simulink model "Table_airbus_v2"  (R2021b)
settings: Solver=VariableStepAuto  StartTime=0.0  StopTime=60*1.5  MaxStep=0.1  RelTol=0.01
undefined symbols (not defined in the file): X, Y, Z
libraries: sm_lib x907, fl_lib x68, nesl_utility x53, sdl_lib x10, simulink x7, ee_lib x7, slpidlib x6, simulink_extras x4
(part 18 of 18)

== system Table_airbus_v2/Modèle mécanique1/Table/table_1_RIGID/x15060_M_01002_Ens_cadre_Default_1_RIGID/x15060_NLM_Ens_guidage_Drylin_N_1_Default_1_RIGID/x15060_NLM_Palier_flottant_21230_2711_1_RIGID ==
  ReferenceFrame : sm_lib/Frames and Transforms/Reference Frame
  Solid : sm_lib/Body Elements/File Solid  ExtGeomFileName=15060-NLM-Palier flottant - 21230-2711_Défaut_sldprt.STL  UnitType=Custom  ExtGeomFileUnits=mm  StepReaderType=HEX  ExportConvexHullGeometry=off  InertiaType=Custom  Mass=0.0034336600000000003  MassUnits=kg  CenterOfMass=[20 6.8081300000000002 0.063214900000000004]  CenterOfMassUnits=mm  MomentsOfInertia=[0.14834700000000001 0.51841599999999999 0.39706900000000001]  MomentsOfInertiaUnits=kg*mm^2  ProductsOfInertia=[-0.00033843699999999997 0 0]  ProductsOfInertiaUnits=kg*mm^2  BasedOnType=Density  Density=1000  DensityUnits=kg/(m^3)  DoExposeReferenceFrame=on  SerializedFrames=<Frames/>  GraphicType=FromGeometry  MarkerShape=Sphere  MarkerSize=10  MarkerSizeUnits=m  GraphicVisPropType=SimpleVisualProperties  GraphicDiffuseColor=[0.792157 0.819608 0.933333]  GraphicSpecularColor=[0.5 0.5 0.5 1.0]  GraphicAmbientColor=[0.15 0.15 0.15 1.0]  GraphicEmissiveColor=[0.0 0.0 0.0 1.0]  GraphicShininess=75  GraphicOpacity=1
  F : PMIOPort  Side=Left
  connections:
  F/RConn1 -- ReferenceFrame/RConn1 -- Solid/RConn1

== system Table_airbus_v2/Modèle mécanique1/Table/table_1_RIGID/x15060_M_01002_Ens_cadre_Default_1_RIGID/x15060_NLM_Ens_guidage_Drylin_N_1_Default_1_RIGID/x15060_NLM_Palier_flottant_21230_2711_2_RIGID ==
  ReferenceFrame : sm_lib/Frames and Transforms/Reference Frame
  Solid : sm_lib/Body Elements/File Solid  ExtGeomFileName=15060-NLM-Palier flottant - 21230-2711_Défaut_sldprt.STL  UnitType=Custom  ExtGeomFileUnits=mm  StepReaderType=HEX  ExportConvexHullGeometry=off  InertiaType=Custom  Mass=0.0034336600000000003  MassUnits=kg  CenterOfMass=[20 6.8081300000000002 0.063214900000000004]  CenterOfMassUnits=mm  MomentsOfInertia=[0.14834700000000001 0.51841599999999999 0.39706900000000001]  MomentsOfInertiaUnits=kg*mm^2  ProductsOfInertia=[-0.00033843699999999997 0 0]  ProductsOfInertiaUnits=kg*mm^2  BasedOnType=Density  Density=1000  DensityUnits=kg/(m^3)  DoExposeReferenceFrame=on  SerializedFrames=<Frames/>  GraphicType=FromGeometry  MarkerShape=Sphere  MarkerSize=10  MarkerSizeUnits=m  GraphicVisPropType=SimpleVisualProperties  GraphicDiffuseColor=[0.792157 0.819608 0.933333]  GraphicSpecularColor=[0.5 0.5 0.5 1.0]  GraphicAmbientColor=[0.15 0.15 0.15 1.0]  GraphicEmissiveColor=[0.0 0.0 0.0 1.0]  GraphicShininess=75  GraphicOpacity=1
  F : PMIOPort  Side=Left
  connections:
  F/RConn1 -- ReferenceFrame/RConn1 -- Solid/RConn1

== system Table_airbus_v2/Modèle mécanique1/Table/table_1_RIGID/x15060_M_01002_Ens_cadre_Default_1_RIGID/x15060_NLM_Ens_guidage_Drylin_N_1_Default_1_RIGID/x15060_NLM_Palier_flottant_21230_2711_3_RIGID ==
  ReferenceFrame : sm_lib/Frames and Transforms/Reference Frame
  Solid : sm_lib/Body Elements/File Solid  ExtGeomFileName=15060-NLM-Palier flottant - 21230-2711_Défaut_sldprt.STL  UnitType=Custom  ExtGeomFileUnits=mm  StepReaderType=HEX  ExportConvexHullGeometry=off  InertiaType=Custom  Mass=0.0034336600000000003  MassUnits=kg  CenterOfMass=[20 6.8081300000000002 0.063214900000000004]  CenterOfMassUnits=mm  MomentsOfInertia=[0.14834700000000001 0.51841599999999999 0.39706900000000001]  MomentsOfInertiaUnits=kg*mm^2  ProductsOfInertia=[-0.00033843699999999997 0 0]  ProductsOfInertiaUnits=kg*mm^2  BasedOnType=Density  Density=1000  DensityUnits=kg/(m^3)  DoExposeReferenceFrame=on  SerializedFrames=<Frames/>  GraphicType=FromGeometry  MarkerShape=Sphere  MarkerSize=10  MarkerSizeUnits=m  GraphicVisPropType=SimpleVisualProperties  GraphicDiffuseColor=[0.792157 0.819608 0.933333]  GraphicSpecularColor=[0.5 0.5 0.5 1.0]  GraphicAmbientColor=[0.15 0.15 0.15 1.0]  GraphicEmissiveColor=[0.0 0.0 0.0 1.0]  GraphicShininess=75  GraphicOpacity=1
  F : PMIOPort  Side=Left
  connections:
  F/RConn1 -- ReferenceFrame/RConn1 -- Solid/RConn1

== system Table_airbus_v2/Modèle mécanique1/Table/table_1_RIGID/x15060_M_01002_Ens_cadre_Default_1_RIGID/x15060_NLM_Ens_guidage_Drylin_N_1_Default_1_RIGID/x15060_NLM_Palier_flottant_21230_2711_4_RIGID ==
  ReferenceFrame : sm_lib/Frames and Transforms/Reference Frame
  Solid : sm_lib/Body Elements/File Solid  ExtGeomFileName=15060-NLM-Palier flottant - 21230-2711_Défaut_sldprt.STL  UnitType=Custom  ExtGeomFileUnits=mm  StepReaderType=HEX  ExportConvexHullGeometry=off  InertiaType=Custom  Mass=0.0034336600000000003  MassUnits=kg  CenterOfMass=[20 6.8081300000000002 0.063214900000000004]  CenterOfMassUnits=mm  MomentsOfInertia=[0.14834700000000001 0.51841599999999999 0.39706900000000001]  MomentsOfInertiaUnits=kg*mm^2  ProductsOfInertia=[-0.00033843699999999997 0 0]  ProductsOfInertiaUnits=kg*mm^2  BasedOnType=Density  Density=1000  DensityUnits=kg/(m^3)  DoExposeReferenceFrame=on  SerializedFrames=<Frames/>  GraphicType=FromGeometry  MarkerShape=Sphere  MarkerSize=10  MarkerSizeUnits=m  GraphicVisPropType=SimpleVisualProperties  GraphicDiffuseColor=[0.792157 0.819608 0.933333]  GraphicSpecularColor=[0.5 0.5 0.5 1.0]  GraphicAmbientColor=[0.15 0.15 0.15 1.0]  GraphicEmissiveColor=[0.0 0.0 0.0 1.0]  GraphicShininess=75  GraphicOpacity=1
  F : PMIOPort  Side=Left
  connections:
  F/RConn1 -- ReferenceFrame/RConn1 -- Solid/RConn1

== system Table_airbus_v2/Modèle mécanique1/Table/table_1_RIGID/x15060_M_01002_Ens_cadre_Default_1_RIGID/x15060_NLM_Ens_guidage_Drylin_N_1_Default_1_RIGID/x15060_NLM_Rail_21230_2730_X_Lgr_1_RIGID ==
  ReferenceFrame : sm_lib/Frames and Transforms/Reference Frame
  Solid : sm_lib/Body Elements/File Solid  ExtGeomFileName=15060-NLM-Rail - 21230-2730 X Lgr._Défaut_sldprt.STL  UnitType=Custom  ExtGeomFileUnits=mm  StepReaderType=HEX  ExportConvexHullGeometry=off  InertiaType=Custom  Mass=0.068416199999999996  MassUnits=kg  CenterOfMass=[390 3.0880299999999998 0]  CenterOfMassUnits=mm  MomentsOfInertia=[4.6660399999999997 2573.8499999999999 2569.9400000000001]  MomentsOfInertiaUnits=kg*mm^2  ProductsOfInertia=[0 0 0]  ProductsOfInertiaUnits=kg*mm^2  BasedOnType=Density  Density=1000  DensityUnits=kg/(m^3)  DoExposeReferenceFrame=on  SerializedFrames=<Frames/>  GraphicType=FromGeometry  MarkerShape=Sphere  MarkerSize=10  MarkerSizeUnits=m  GraphicVisPropType=SimpleVisualProperties  GraphicDiffuseColor=[0.792157 0.819608 0.933333]  GraphicSpecularColor=[0.5 0.5 0.5 1.0]  GraphicAmbientColor=[0.15 0.15 0.15 1.0]  GraphicEmissiveColor=[0.0 0.0 0.0 1.0]  GraphicShininess=75  GraphicOpacity=1
  F : PMIOPort  Side=Left
  connections:
  F/RConn1 -- ReferenceFrame/RConn1 -- Solid/RConn1

== system Table_airbus_v2/Modèle mécanique1/Table/table_1_RIGID/x15060_M_01002_Ens_cadre_Default_1_RIGID/x15060_NLM_Ens_guidage_Drylin_N_1_Default_2_RIGID/x15060_NLM_Palier_flottant_21230_2711_1_RIGID ==
  ReferenceFrame : sm_lib/Frames and Transforms/Reference Frame
  Solid : sm_lib/Body Elements/File Solid  ExtGeomFileName=15060-NLM-Palier flottant - 21230-2711_Défaut_sldprt.STL  UnitType=Custom  ExtGeomFileUnits=mm  StepReaderType=HEX  ExportConvexHullGeometry=off  InertiaType=Custom  Mass=0.0034336600000000003  MassUnits=kg  CenterOfMass=[20 6.8081300000000002 0.063214900000000004]  CenterOfMassUnits=mm  MomentsOfInertia=[0.14834700000000001 0.51841599999999999 0.39706900000000001]  MomentsOfInertiaUnits=kg*mm^2  ProductsOfInertia=[-0.00033843699999999997 0 0]  ProductsOfInertiaUnits=kg*mm^2  BasedOnType=Density  Density=1000  DensityUnits=kg/(m^3)  DoExposeReferenceFrame=on  SerializedFrames=<Frames/>  GraphicType=FromGeometry  MarkerShape=Sphere  MarkerSize=10  MarkerSizeUnits=m  GraphicVisPropType=SimpleVisualProperties  GraphicDiffuseColor=[0.792157 0.819608 0.933333]  GraphicSpecularColor=[0.5 0.5 0.5 1.0]  GraphicAmbientColor=[0.15 0.15 0.15 1.0]  GraphicEmissiveColor=[0.0 0.0 0.0 1.0]  GraphicShininess=75  GraphicOpacity=1
  F : PMIOPort  Side=Left
  connections:
  F/RConn1 -- ReferenceFrame/RConn1 -- Solid/RConn1

== system Table_airbus_v2/Modèle mécanique1/Table/table_1_RIGID/x15060_M_01002_Ens_cadre_Default_1_RIGID/x15060_NLM_Ens_guidage_Drylin_N_1_Default_2_RIGID/x15060_NLM_Palier_flottant_21230_2711_2_RIGID ==
  ReferenceFrame : sm_lib/Frames and Transforms/Reference Frame
  Solid : sm_lib/Body Elements/File Solid  ExtGeomFileName=15060-NLM-Palier flottant - 21230-2711_Défaut_sldprt.STL  UnitType=Custom  ExtGeomFileUnits=mm  StepReaderType=HEX  ExportConvexHullGeometry=off  InertiaType=Custom  Mass=0.0034336600000000003  MassUnits=kg  CenterOfMass=[20 6.8081300000000002 0.063214900000000004]  CenterOfMassUnits=mm  MomentsOfInertia=[0.14834700000000001 0.51841599999999999 0.39706900000000001]  MomentsOfInertiaUnits=kg*mm^2  ProductsOfInertia=[-0.00033843699999999997 0 0]  ProductsOfInertiaUnits=kg*mm^2  BasedOnType=Density  Density=1000  DensityUnits=kg/(m^3)  DoExposeReferenceFrame=on  SerializedFrames=<Frames/>  GraphicType=FromGeometry  MarkerShape=Sphere  MarkerSize=10  MarkerSizeUnits=m  GraphicVisPropType=SimpleVisualProperties  GraphicDiffuseColor=[0.792157 0.819608 0.933333]  GraphicSpecularColor=[0.5 0.5 0.5 1.0]  GraphicAmbientColor=[0.15 0.15 0.15 1.0]  GraphicEmissiveColor=[0.0 0.0 0.0 1.0]  GraphicShininess=75  GraphicOpacity=1
  F : PMIOPort  Side=Left
  connections:
  F/RConn1 -- ReferenceFrame/RConn1 -- Solid/RConn1

== system Table_airbus_v2/Modèle mécanique1/Table/table_1_RIGID/x15060_M_01002_Ens_cadre_Default_1_RIGID/x15060_NLM_Ens_guidage_Drylin_N_1_Default_2_RIGID/x15060_NLM_Palier_flottant_21230_2711_3_RIGID ==
  ReferenceFrame : sm_lib/Frames and Transforms/Reference Frame
  Solid : sm_lib/Body Elements/File Solid  ExtGeomFileName=15060-NLM-Palier flottant - 21230-2711_Défaut_sldprt.STL  UnitType=Custom  ExtGeomFileUnits=mm  StepReaderType=HEX  ExportConvexHullGeometry=off  InertiaType=Custom  Mass=0.0034336600000000003  MassUnits=kg  CenterOfMass=[20 6.8081300000000002 0.063214900000000004]  CenterOfMassUnits=mm  MomentsOfInertia=[0.14834700000000001 0.51841599999999999 0.39706900000000001]  MomentsOfInertiaUnits=kg*mm^2  ProductsOfInertia=[-0.00033843699999999997 0 0]  ProductsOfInertiaUnits=kg*mm^2  BasedOnType=Density  Density=1000  DensityUnits=kg/(m^3)  DoExposeReferenceFrame=on  SerializedFrames=<Frames/>  GraphicType=FromGeometry  MarkerShape=Sphere  MarkerSize=10  MarkerSizeUnits=m  GraphicVisPropType=SimpleVisualProperties  GraphicDiffuseColor=[0.792157 0.819608 0.933333]  GraphicSpecularColor=[0.5 0.5 0.5 1.0]  GraphicAmbientColor=[0.15 0.15 0.15 1.0]  GraphicEmissiveColor=[0.0 0.0 0.0 1.0]  GraphicShininess=75  GraphicOpacity=1
  F : PMIOPort  Side=Left
  connections:
  F/RConn1 -- ReferenceFrame/RConn1 -- Solid/RConn1

== system Table_airbus_v2/Modèle mécanique1/Table/table_1_RIGID/x15060_M_01002_Ens_cadre_Default_1_RIGID/x15060_NLM_Ens_guidage_Drylin_N_1_Default_2_RIGID/x15060_NLM_Palier_flottant_21230_2711_4_RIGID ==
  ReferenceFrame : sm_lib/Frames and Transforms/Reference Frame
  Solid : sm_lib/Body Elements/File Solid  ExtGeomFileName=15060-NLM-Palier flottant - 21230-2711_Défaut_sldprt.STL  UnitType=Custom  ExtGeomFileUnits=mm  StepReaderType=HEX  ExportConvexHullGeometry=off  InertiaType=Custom  Mass=0.0034336600000000003  MassUnits=kg  CenterOfMass=[20 6.8081300000000002 0.063214900000000004]  CenterOfMassUnits=mm  MomentsOfInertia=[0.14834700000000001 0.51841599999999999 0.39706900000000001]  MomentsOfInertiaUnits=kg*mm^2  ProductsOfInertia=[-0.00033843699999999997 0 0]  ProductsOfInertiaUnits=kg*mm^2  BasedOnType=Density  Density=1000  DensityUnits=kg/(m^3)  DoExposeReferenceFrame=on  SerializedFrames=<Frames/>  GraphicType=FromGeometry  MarkerShape=Sphere  MarkerSize=10  MarkerSizeUnits=m  GraphicVisPropType=SimpleVisualProperties  GraphicDiffuseColor=[0.792157 0.819608 0.933333]  GraphicSpecularColor=[0.5 0.5 0.5 1.0]  GraphicAmbientColor=[0.15 0.15 0.15 1.0]  GraphicEmissiveColor=[0.0 0.0 0.0 1.0]  GraphicShininess=75  GraphicOpacity=1
  F : PMIOPort  Side=Left
  connections:
  F/RConn1 -- ReferenceFrame/RConn1 -- Solid/RConn1

== system Table_airbus_v2/Modèle mécanique1/Table/table_1_RIGID/x15060_M_01002_Ens_cadre_Default_1_RIGID/x15060_NLM_Ens_guidage_Drylin_N_1_Default_2_RIGID/x15060_NLM_Rail_21230_2730_X_Lgr_1_RIGID ==
  ReferenceFrame : sm_lib/Frames and Transforms/Reference Frame
  Solid : sm_lib/Body Elements/File Solid  ExtGeomFileName=15060-NLM-Rail - 21230-2730 X Lgr._Défaut_sldprt.STL  UnitType=Custom  ExtGeomFileUnits=mm  StepReaderType=HEX  ExportConvexHullGeometry=off  InertiaType=Custom  Mass=0.068416199999999996  MassUnits=kg  CenterOfMass=[390 3.0880299999999998 0]  CenterOfMassUnits=mm  MomentsOfInertia=[4.6660399999999997 2573.8499999999999 2569.9400000000001]  MomentsOfInertiaUnits=kg*mm^2  ProductsOfInertia=[0 0 0]  ProductsOfInertiaUnits=kg*mm^2  BasedOnType=Density  Density=1000  DensityUnits=kg/(m^3)  DoExposeReferenceFrame=on  SerializedFrames=<Frames/>  GraphicType=FromGeometry  MarkerShape=Sphere  MarkerSize=10  MarkerSizeUnits=m  GraphicVisPropType=SimpleVisualProperties  GraphicDiffuseColor=[0.792157 0.819608 0.933333]  GraphicSpecularColor=[0.5 0.5 0.5 1.0]  GraphicAmbientColor=[0.15 0.15 0.15 1.0]  GraphicEmissiveColor=[0.0 0.0 0.0 1.0]  GraphicShininess=75  GraphicOpacity=1
  F : PMIOPort  Side=Left
  connections:
  F/RConn1 -- ReferenceFrame/RConn1 -- Solid/RConn1

== system Table_airbus_v2/Modèle mécanique1/Table/table_1_RIGID/x15060_M_01002_Ens_cadre_Default_1_RIGID/x15060_NLM_Ens_guidage_Drylin_N_1_Default_3_RIGID/x15060_NLM_Palier_flottant_21230_2711_1_RIGID ==
  ReferenceFrame : sm_lib/Frames and Transforms/Reference Frame
  Solid : sm_lib/Body Elements/File Solid  ExtGeomFileName=15060-NLM-Palier flottant - 21230-2711_Défaut_sldprt.STL  UnitType=Custom  ExtGeomFileUnits=mm  StepReaderType=HEX  ExportConvexHullGeometry=off  InertiaType=Custom  Mass=0.0034336600000000003  MassUnits=kg  CenterOfMass=[20 6.8081300000000002 0.063214900000000004]  CenterOfMassUnits=mm  MomentsOfInertia=[0.14834700000000001 0.51841599999999999 0.39706900000000001]  MomentsOfInertiaUnits=kg*mm^2  ProductsOfInertia=[-0.00033843699999999997 0 0]  ProductsOfInertiaUnits=kg*mm^2  BasedOnType=Density  Density=1000  DensityUnits=kg/(m^3)  DoExposeReferenceFrame=on  SerializedFrames=<Frames/>  GraphicType=FromGeometry  MarkerShape=Sphere  MarkerSize=10  MarkerSizeUnits=m  GraphicVisPropType=SimpleVisualProperties  GraphicDiffuseColor=[0.792157 0.819608 0.933333]  GraphicSpecularColor=[0.5 0.5 0.5 1.0]  GraphicAmbientColor=[0.15 0.15 0.15 1.0]  GraphicEmissiveColor=[0.0 0.0 0.0 1.0]  GraphicShininess=75  GraphicOpacity=1
  F : PMIOPort  Side=Left
  connections:
  F/RConn1 -- ReferenceFrame/RConn1 -- Solid/RConn1

== system Table_airbus_v2/Modèle mécanique1/Table/table_1_RIGID/x15060_M_01002_Ens_cadre_Default_1_RIGID/x15060_NLM_Ens_guidage_Drylin_N_1_Default_3_RIGID/x15060_NLM_Palier_flottant_21230_2711_2_RIGID ==
  ReferenceFrame : sm_lib/Frames and Transforms/Reference Frame
  Solid : sm_lib/Body Elements/File Solid  ExtGeomFileName=15060-NLM-Palier flottant - 21230-2711_Défaut_sldprt.STL  UnitType=Custom  ExtGeomFileUnits=mm  StepReaderType=HEX  ExportConvexHullGeometry=off  InertiaType=Custom  Mass=0.0034336600000000003  MassUnits=kg  CenterOfMass=[20 6.8081300000000002 0.063214900000000004]  CenterOfMassUnits=mm  MomentsOfInertia=[0.14834700000000001 0.51841599999999999 0.39706900000000001]  MomentsOfInertiaUnits=kg*mm^2  ProductsOfInertia=[-0.00033843699999999997 0 0]  ProductsOfInertiaUnits=kg*mm^2  BasedOnType=Density  Density=1000  DensityUnits=kg/(m^3)  DoExposeReferenceFrame=on  SerializedFrames=<Frames/>  GraphicType=FromGeometry  MarkerShape=Sphere  MarkerSize=10  MarkerSizeUnits=m  GraphicVisPropType=SimpleVisualProperties  GraphicDiffuseColor=[0.792157 0.819608 0.933333]  GraphicSpecularColor=[0.5 0.5 0.5 1.0]  GraphicAmbientColor=[0.15 0.15 0.15 1.0]  GraphicEmissiveColor=[0.0 0.0 0.0 1.0]  GraphicShininess=75  GraphicOpacity=1
  F : PMIOPort  Side=Left
  connections:
  F/RConn1 -- ReferenceFrame/RConn1 -- Solid/RConn1

== system Table_airbus_v2/Modèle mécanique1/Table/table_1_RIGID/x15060_M_01002_Ens_cadre_Default_1_RIGID/x15060_NLM_Ens_guidage_Drylin_N_1_Default_3_RIGID/x15060_NLM_Palier_flottant_21230_2711_3_RIGID ==
  ReferenceFrame : sm_lib/Frames and Transforms/Reference Frame
  Solid : sm_lib/Body Elements/File Solid  ExtGeomFileName=15060-NLM-Palier flottant - 21230-2711_Défaut_sldprt.STL  UnitType=Custom  ExtGeomFileUnits=mm  StepReaderType=HEX  ExportConvexHullGeometry=off  InertiaType=Custom  Mass=0.0034336600000000003  MassUnits=kg  CenterOfMass=[20 6.8081300000000002 0.063214900000000004]  CenterOfMassUnits=mm  MomentsOfInertia=[0.14834700000000001 0.51841599999999999 0.39706900000000001]  MomentsOfInertiaUnits=kg*mm^2  ProductsOfInertia=[-0.00033843699999999997 0 0]  ProductsOfInertiaUnits=kg*mm^2  BasedOnType=Density  Density=1000  DensityUnits=kg/(m^3)  DoExposeReferenceFrame=on  SerializedFrames=<Frames/>  GraphicType=FromGeometry  MarkerShape=Sphere  MarkerSize=10  MarkerSizeUnits=m  GraphicVisPropType=SimpleVisualProperties  GraphicDiffuseColor=[0.792157 0.819608 0.933333]  GraphicSpecularColor=[0.5 0.5 0.5 1.0]  GraphicAmbientColor=[0.15 0.15 0.15 1.0]  GraphicEmissiveColor=[0.0 0.0 0.0 1.0]  GraphicShininess=75  GraphicOpacity=1
  F : PMIOPort  Side=Left
  connections:
  F/RConn1 -- ReferenceFrame/RConn1 -- Solid/RConn1

== system Table_airbus_v2/Modèle mécanique1/Table/table_1_RIGID/x15060_M_01002_Ens_cadre_Default_1_RIGID/x15060_NLM_Ens_guidage_Drylin_N_1_Default_3_RIGID/x15060_NLM_Palier_flottant_21230_2711_4_RIGID ==
  ReferenceFrame : sm_lib/Frames and Transforms/Reference Frame
  Solid : sm_lib/Body Elements/File Solid  ExtGeomFileName=15060-NLM-Palier flottant - 21230-2711_Défaut_sldprt.STL  UnitType=Custom  ExtGeomFileUnits=mm  StepReaderType=HEX  ExportConvexHullGeometry=off  InertiaType=Custom  Mass=0.0034336600000000003  MassUnits=kg  CenterOfMass=[20 6.8081300000000002 0.063214900000000004]  CenterOfMassUnits=mm  MomentsOfInertia=[0.14834700000000001 0.51841599999999999 0.39706900000000001]  MomentsOfInertiaUnits=kg*mm^2  ProductsOfInertia=[-0.00033843699999999997 0 0]  ProductsOfInertiaUnits=kg*mm^2  BasedOnType=Density  Density=1000  DensityUnits=kg/(m^3)  DoExposeReferenceFrame=on  SerializedFrames=<Frames/>  GraphicType=FromGeometry  MarkerShape=Sphere  MarkerSize=10  MarkerSizeUnits=m  GraphicVisPropType=SimpleVisualProperties  GraphicDiffuseColor=[0.792157 0.819608 0.933333]  GraphicSpecularColor=[0.5 0.5 0.5 1.0]  GraphicAmbientColor=[0.15 0.15 0.15 1.0]  GraphicEmissiveColor=[0.0 0.0 0.0 1.0]  GraphicShininess=75  GraphicOpacity=1
  F : PMIOPort  Side=Left
  connections:
  F/RConn1 -- ReferenceFrame/RConn1 -- Solid/RConn1

== system Table_airbus_v2/Modèle mécanique1/Table/table_1_RIGID/x15060_M_01002_Ens_cadre_Default_1_RIGID/x15060_NLM_Ens_guidage_Drylin_N_1_Default_3_RIGID/x15060_NLM_Rail_21230_2730_X_Lgr_1_RIGID ==
  ReferenceFrame : sm_lib/Frames and Transforms/Reference Frame
  Solid : sm_lib/Body Elements/File Solid  ExtGeomFileName=15060-NLM-Rail - 21230-2730 X Lgr._Défaut_sldprt.STL  UnitType=Custom  ExtGeomFileUnits=mm  StepReaderType=HEX  ExportConvexHullGeometry=off  InertiaType=Custom  Mass=0.068416199999999996  MassUnits=kg  CenterOfMass=[390 3.0880299999999998 0]  CenterOfMassUnits=mm  MomentsOfInertia=[4.6660399999999997 2573.8499999999999 2569.9400000000001]  MomentsOfInertiaUnits=kg*mm^2  ProductsOfInertia=[0 0 0]  ProductsOfInertiaUnits=kg*mm^2  BasedOnType=Density  Density=1000  DensityUnits=kg/(m^3)  DoExposeReferenceFrame=on  SerializedFrames=<Frames/>  GraphicType=FromGeometry  MarkerShape=Sphere  MarkerSize=10  MarkerSizeUnits=m  GraphicVisPropType=SimpleVisualProperties  GraphicDiffuseColor=[0.792157 0.819608 0.933333]  GraphicSpecularColor=[0.5 0.5 0.5 1.0]  GraphicAmbientColor=[0.15 0.15 0.15 1.0]  GraphicEmissiveColor=[0.0 0.0 0.0 1.0]  GraphicShininess=75  GraphicOpacity=1
  F : PMIOPort  Side=Left
  connections:
  F/RConn1 -- ReferenceFrame/RConn1 -- Solid/RConn1

== system Table_airbus_v2/Modèle mécanique1/Table/table_1_RIGID/x15060_M_01002_Ens_cadre_Default_1_RIGID/x15060_NLM_Ens_guidage_Drylin_N_1_Default_4_RIGID/x15060_NLM_Palier_flottant_21230_2711_1_RIGID ==
  ReferenceFrame : sm_lib/Frames and Transforms/Reference Frame
  Solid : sm_lib/Body Elements/File Solid  ExtGeomFileName=15060-NLM-Palier flottant - 21230-2711_Défaut_sldprt.STL  UnitType=Custom  ExtGeomFileUnits=mm  StepReaderType=HEX  ExportConvexHullGeometry=off  InertiaType=Custom  Mass=0.0034336600000000003  MassUnits=kg  CenterOfMass=[20 6.8081300000000002 0.063214900000000004]  CenterOfMassUnits=mm  MomentsOfInertia=[0.14834700000000001 0.51841599999999999 0.39706900000000001]  MomentsOfInertiaUnits=kg*mm^2  ProductsOfInertia=[-0.00033843699999999997 0 0]  ProductsOfInertiaUnits=kg*mm^2  BasedOnType=Density  Density=1000  DensityUnits=kg/(m^3)  DoExposeReferenceFrame=on  SerializedFrames=<Frames/>  GraphicType=FromGeometry  MarkerShape=Sphere  MarkerSize=10  MarkerSizeUnits=m  GraphicVisPropType=SimpleVisualProperties  GraphicDiffuseColor=[0.792157 0.819608 0.933333]  GraphicSpecularColor=[0.5 0.5 0.5 1.0]  GraphicAmbientColor=[0.15 0.15 0.15 1.0]  GraphicEmissiveColor=[0.0 0.0 0.0 1.0]  GraphicShininess=75  GraphicOpacity=1
  F : PMIOPort  Side=Left
  connections:
  F/RConn1 -- ReferenceFrame/RConn1 -- Solid/RConn1

== system Table_airbus_v2/Modèle mécanique1/Table/table_1_RIGID/x15060_M_01002_Ens_cadre_Default_1_RIGID/x15060_NLM_Ens_guidage_Drylin_N_1_Default_4_RIGID/x15060_NLM_Palier_flottant_21230_2711_2_RIGID ==
  ReferenceFrame : sm_lib/Frames and Transforms/Reference Frame
  Solid : sm_lib/Body Elements/File Solid  ExtGeomFileName=15060-NLM-Palier flottant - 21230-2711_Défaut_sldprt.STL  UnitType=Custom  ExtGeomFileUnits=mm  StepReaderType=HEX  ExportConvexHullGeometry=off  InertiaType=Custom  Mass=0.0034336600000000003  MassUnits=kg  CenterOfMass=[20 6.8081300000000002 0.063214900000000004]  CenterOfMassUnits=mm  MomentsOfInertia=[0.14834700000000001 0.51841599999999999 0.39706900000000001]  MomentsOfInertiaUnits=kg*mm^2  ProductsOfInertia=[-0.00033843699999999997 0 0]  ProductsOfInertiaUnits=kg*mm^2  BasedOnType=Density  Density=1000  DensityUnits=kg/(m^3)  DoExposeReferenceFrame=on  SerializedFrames=<Frames/>  GraphicType=FromGeometry  MarkerShape=Sphere  MarkerSize=10  MarkerSizeUnits=m  GraphicVisPropType=SimpleVisualProperties  GraphicDiffuseColor=[0.792157 0.819608 0.933333]  GraphicSpecularColor=[0.5 0.5 0.5 1.0]  GraphicAmbientColor=[0.15 0.15 0.15 1.0]  GraphicEmissiveColor=[0.0 0.0 0.0 1.0]  GraphicShininess=75  GraphicOpacity=1
  F : PMIOPort  Side=Left
  connections:
  F/RConn1 -- ReferenceFrame/RConn1 -- Solid/RConn1

== system Table_airbus_v2/Modèle mécanique1/Table/table_1_RIGID/x15060_M_01002_Ens_cadre_Default_1_RIGID/x15060_NLM_Ens_guidage_Drylin_N_1_Default_4_RIGID/x15060_NLM_Palier_flottant_21230_2711_3_RIGID ==
  ReferenceFrame : sm_lib/Frames and Transforms/Reference Frame
  Solid : sm_lib/Body Elements/File Solid  ExtGeomFileName=15060-NLM-Palier flottant - 21230-2711_Défaut_sldprt.STL  UnitType=Custom  ExtGeomFileUnits=mm  StepReaderType=HEX  ExportConvexHullGeometry=off  InertiaType=Custom  Mass=0.0034336600000000003  MassUnits=kg  CenterOfMass=[20 6.8081300000000002 0.063214900000000004]  CenterOfMassUnits=mm  MomentsOfInertia=[0.14834700000000001 0.51841599999999999 0.39706900000000001]  MomentsOfInertiaUnits=kg*mm^2  ProductsOfInertia=[-0.00033843699999999997 0 0]  ProductsOfInertiaUnits=kg*mm^2  BasedOnType=Density  Density=1000  DensityUnits=kg/(m^3)  DoExposeReferenceFrame=on  SerializedFrames=<Frames/>  GraphicType=FromGeometry  MarkerShape=Sphere  MarkerSize=10  MarkerSizeUnits=m  GraphicVisPropType=SimpleVisualProperties  GraphicDiffuseColor=[0.792157 0.819608 0.933333]  GraphicSpecularColor=[0.5 0.5 0.5 1.0]  GraphicAmbientColor=[0.15 0.15 0.15 1.0]  GraphicEmissiveColor=[0.0 0.0 0.0 1.0]  GraphicShininess=75  GraphicOpacity=1
  F : PMIOPort  Side=Left
  connections:
  F/RConn1 -- ReferenceFrame/RConn1 -- Solid/RConn1

== system Table_airbus_v2/Modèle mécanique1/Table/table_1_RIGID/x15060_M_01002_Ens_cadre_Default_1_RIGID/x15060_NLM_Ens_guidage_Drylin_N_1_Default_4_RIGID/x15060_NLM_Palier_flottant_21230_2711_4_RIGID ==
  ReferenceFrame : sm_lib/Frames and Transforms/Reference Frame
  Solid : sm_lib/Body Elements/File Solid  ExtGeomFileName=15060-NLM-Palier flottant - 21230-2711_Défaut_sldprt.STL  UnitType=Custom  ExtGeomFileUnits=mm  StepReaderType=HEX  ExportConvexHullGeometry=off  InertiaType=Custom  Mass=0.0034336600000000003  MassUnits=kg  CenterOfMass=[20 6.8081300000000002 0.063214900000000004]  CenterOfMassUnits=mm  MomentsOfInertia=[0.14834700000000001 0.51841599999999999 0.39706900000000001]  MomentsOfInertiaUnits=kg*mm^2  ProductsOfInertia=[-0.00033843699999999997 0 0]  ProductsOfInertiaUnits=kg*mm^2  BasedOnType=Density  Density=1000  DensityUnits=kg/(m^3)  DoExposeReferenceFrame=on  SerializedFrames=<Frames/>  GraphicType=FromGeometry  MarkerShape=Sphere  MarkerSize=10  MarkerSizeUnits=m  GraphicVisPropType=SimpleVisualProperties  GraphicDiffuseColor=[0.792157 0.819608 0.933333]  GraphicSpecularColor=[0.5 0.5 0.5 1.0]  GraphicAmbientColor=[0.15 0.15 0.15 1.0]  GraphicEmissiveColor=[0.0 0.0 0.0 1.0]  GraphicShininess=75  GraphicOpacity=1
  F : PMIOPort  Side=Left
  connections:
  F/RConn1 -- ReferenceFrame/RConn1 -- Solid/RConn1

== system Table_airbus_v2/Modèle mécanique1/Table/table_1_RIGID/x15060_M_01002_Ens_cadre_Default_1_RIGID/x15060_NLM_Ens_guidage_Drylin_N_1_Default_4_RIGID/x15060_NLM_Rail_21230_2730_X_Lgr_1_RIGID ==
  ReferenceFrame : sm_lib/Frames and Transforms/Reference Frame
  Solid : sm_lib/Body Elements/File Solid  ExtGeomFileName=15060-NLM-Rail - 21230-2730 X Lgr._Défaut_sldprt.STL  UnitType=Custom  ExtGeomFileUnits=mm  StepReaderType=HEX  ExportConvexHullGeometry=off  InertiaType=Custom  Mass=0.068416199999999996  MassUnits=kg  CenterOfMass=[390 3.0880299999999998 0]  CenterOfMassUnits=mm  MomentsOfInertia=[4.6660399999999997 2573.8499999999999 2569.9400000000001]  MomentsOfInertiaUnits=kg*mm^2  ProductsOfInertia=[0 0 0]  ProductsOfInertiaUnits=kg*mm^2  BasedOnType=Density  Density=1000  DensityUnits=kg/(m^3)  DoExposeReferenceFrame=on  SerializedFrames=<Frames/>  GraphicType=FromGeometry  MarkerShape=Sphere  MarkerSize=10  MarkerSizeUnits=m  GraphicVisPropType=SimpleVisualProperties  GraphicDiffuseColor=[0.792157 0.819608 0.933333]  GraphicSpecularColor=[0.5 0.5 0.5 1.0]  GraphicAmbientColor=[0.15 0.15 0.15 1.0]  GraphicEmissiveColor=[0.0 0.0 0.0 1.0]  GraphicShininess=75  GraphicOpacity=1
  F : PMIOPort  Side=Left
  connections:
  F/RConn1 -- ReferenceFrame/RConn1 -- Solid/RConn1

== system Table_airbus_v2/Modèle mécanique1/Table/table_1_RIGID/x15060_M_01014_Ens_plateau_Default_1_RIGID/x15060_M_01003_Ens_structure_plateau_Default_1_RIGID/x15060_ITEM_Kit_Equerre_8_40x40_Zn_0_0_411_15_AA_DEFAULT_1_RIGI ==
  ReferenceFrame : sm_lib/Frames and Transforms/Reference Frame
  Solid : sm_lib/Body Elements/File Solid  ExtGeomFileName=15060-ITEM-Kit Equerre 8 40x40 Zn - 0.0.411.15_AA - DEFAULT_Défaut_sldprt.STL  UnitType=Custom  ExtGeomFileUnits=mm  StepReaderType=HEX  ExportConvexHullGeometry=off  InertiaType=Custom  Mass=0.010278799999999999  MassUnits=kg  CenterOfMass=[11.6701 11.6701 0]  CenterOfMassUnits=mm  MomentsOfInertia=[3.3914200000000001 3.3914200000000001 2.6288999999999998]  MomentsOfInertiaUnits=kg*mm^2  ProductsOfInertia=[0 0 -0.71321800000000002]  ProductsOfInertiaUnits=kg*mm^2  BasedOnType=Density  Density=1000  DensityUnits=kg/(m^3)  DoExposeReferenceFrame=on  SerializedFrames=<Frames/>  GraphicType=FromGeometry  MarkerShape=Sphere  MarkerSize=10  MarkerSizeUnits=m  GraphicVisPropType=SimpleVisualProperties  GraphicDiffuseColor=[0.792157 0.819608 0.933333]  GraphicSpecularColor=[0.5 0.5 0.5 1.0]  GraphicAmbientColor=[0.15 0.15 0.15 1.0]  GraphicEmissiveColor=[0.0 0.0 0.0 1.0]  GraphicShininess=75  GraphicOpacity=1
  F : PMIOPort  Side=Left
  connections:
  F/RConn1 -- ReferenceFrame/RConn1 -- Solid/RConn1

== system Table_airbus_v2/Modèle mécanique1/Table/table_1_RIGID/x15060_M_01014_Ens_plateau_Default_1_RIGID/x15060_M_01003_Ens_structure_plateau_Default_1_RIGID/x15060_ITEM_Kit_Equerre_8_80x80_Zn_0_0_411_32_AA_DEFAULT_1_RIGI ==
  ReferenceFrame : sm_lib/Frames and Transforms/Reference Frame
  Solid : sm_lib/Body Elements/File Solid  ExtGeomFileName=15060-ITEM-Kit Equerre 8 80x80 Zn - 0.0.411.32_AA - DEFAULT_Défaut_sldprt.STL  UnitType=Custom  ExtGeomFileUnits=mm  StepReaderType=HEX  ExportConvexHullGeometry=off  InertiaType=Custom  Mass=0.078431600000000004  MassUnits=kg  CenterOfMass=[23.9558 23.9558 0]  CenterOfMassUnits=mm  MomentsOfInertia=[57.169000000000004 57.169000000000004 76.38539999999999]  MomentsOfInertiaUnits=kg*mm^2  ProductsOfInertia=[0 0 -20.189700000000002]  ProductsOfInertiaUnits=kg*mm^2  BasedOnType=Density  Density=1000  DensityUnits=kg/(m^3)  DoExposeReferenceFrame=on  SerializedFrames=<Frames/>  GraphicType=FromGeometry  MarkerShape=Sphere  MarkerSize=10  MarkerSizeUnits=m  GraphicVisPropType=SimpleVisualProperties  GraphicDiffuseColor=[0.898039 0.917647 0.929412]  GraphicSpecularColor=[0.5 0.5 0.5 1.0]  GraphicAmbientColor=[0.15 0.15 0.15 1.0]  GraphicEmissiveColor=[0.0 0.0 0.0 1.0]  GraphicShininess=75  GraphicOpacity=1
  F : PMIOPort  Side=Left
  connections:
  F/RConn1 -- ReferenceFrame/RConn1 -- Solid/RConn1

== system Table_airbus_v2/Modèle mécanique1/Table/table_1_RIGID/x15060_M_01014_Ens_plateau_Default_1_RIGID/x15060_M_01003_Ens_structure_plateau_Default_1_RIGID/x15060_ITEM_Kit_Equerre_8_80x80_Zn_0_0_411_32_AA_DEFAULT_2_RIGI ==
  ReferenceFrame : sm_lib/Frames and Transforms/Reference Frame
  Solid : sm_lib/Body Elements/File Solid  ExtGeomFileName=15060-ITEM-Kit Equerre 8 80x80 Zn - 0.0.411.32_AA - DEFAULT_Défaut_sldprt.STL  UnitType=Custom  ExtGeomFileUnits=mm  StepReaderType=HEX  ExportConvexHullGeometry=off  InertiaType=Custom  Mass=0.078431600000000004  MassUnits=kg  CenterOfMass=[23.9558 23.9558 0]  CenterOfMassUnits=mm  MomentsOfInertia=[57.169000000000004 57.169000000000004 76.38539999999999]  MomentsOfInertiaUnits=kg*mm^2  ProductsOfInertia=[0 0 -20.189700000000002]  ProductsOfInertiaUnits=kg*mm^2  BasedOnType=Density  Density=1000  DensityUnits=kg/(m^3)  DoExposeReferenceFrame=on  SerializedFrames=<Frames/>  GraphicType=FromGeometry  MarkerShape=Sphere  MarkerSize=10  MarkerSizeUnits=m  GraphicVisPropType=SimpleVisualProperties  GraphicDiffuseColor=[0.898039 0.917647 0.929412]  GraphicSpecularColor=[0.5 0.5 0.5 1.0]  GraphicAmbientColor=[0.15 0.15 0.15 1.0]  GraphicEmissiveColor=[0.0 0.0 0.0 1.0]  GraphicShininess=75  GraphicOpacity=1
  F : PMIOPort  Side=Left
  connections:
  F/RConn1 -- ReferenceFrame/RConn1 -- Solid/RConn1

== system Table_airbus_v2/Modèle mécanique1/Table/table_1_RIGID/x15060_M_01014_Ens_plateau_Default_1_RIGID/x15060_M_01003_Ens_structure_plateau_Default_1_RIGID/x15060_M_01021_Plateau_en_profil_alu_40x40_AA_DEFAULT_Brut_dusi ==
  ReferenceFrame : sm_lib/Frames and Transforms/Reference Frame
  Solid : sm_lib/Body Elements/File Solid  ExtGeomFileName=15060-M-01021-Plateau en profil alu 40x40_AA - DEFAULT_Brut d''usinage__Défaut_sldprt.STL  UnitType=Custom  ExtGeomFileUnits=mm  StepReaderType=HEX  ExportConvexHullGeometry=off  InertiaType=Custom  Mass=25.0426  MassUnits=kg  CenterOfMass=[24.433300000000003 -0.24912499999999999 -1.82218e-07]  CenterOfMassUnits=mm  MomentsOfInertia=[2090520.0000000002 8521360 10604200]  MomentsOfInertiaUnits=kg*mm^2  ProductsOfInertia=[0.00116004 0.0095347399999999999 152.37299999999999]  ProductsOfInertiaUnits=kg*mm^2  BasedOnType=Density  Density=1000  DensityUnits=kg/(m^3)  DoExposeReferenceFrame=on  SerializedFrames=<Frames/>  GraphicType=FromGeometry  MarkerShape=Sphere  MarkerSize=10  MarkerSizeUnits=m  GraphicVisPropType=SimpleVisualProperties  GraphicDiffuseColor=[0.898039 0.917647 0.929412]  GraphicSpecularColor=[0.5 0.5 0.5 1.0]  GraphicAmbientColor=[0.15 0.15 0.15 1.0]  GraphicEmissiveColor=[0.0 0.0 0.0 1.0]  GraphicShininess=75  GraphicOpacity=1
  F : PMIOPort  Side=Left
  connections:
  F/RConn1 -- ReferenceFrame/RConn1 -- Solid/RConn1

== stateflow chart Table_airbus_v2/Chart ==
  state H0
    H_dem=250;
    I_dem=0;
  state H01
    H_dem=600;
    I_dem=0;
  state H07
  state H08
  state H02
    H_dem=600;
    I_dem=5;
  state H03
    H_dem=600;
    I_dem=-20;
  state H09
  state H04
    H_dem=600;
    I_dem=0;
  state H010
  state H05
    H_dem=400;
    I_dem=0;
  state H011
  state H06
    H_dem=250;
    I_dem=0;
  (default) -> H0
  H0 -> H01 : after(1,sec)
  H01 -> H07 : [Flev==1]
  H07 -> H02 : after(5,sec)
  H02 -> H08 : [Finc==1]
  H08 -> H03 : after(5,sec)
  H03 -> H09 : [Finc==1]
  H09 -> H04 : after(5,sec)
  H04 -> H010 : [Finc==1]
  H010 -> H05 : after(5,sec)
  H05 -> H011 : [Flev==1]
  H011 -> H06 : after(5,sec)
  data: H_dem output; I_dem output; Flev input; Finc input

== matlab function Table_airbus_v2/Ordinateur/MATLAB Function6 ==
  data: course_m input; hauteur output
function hauteur = fcn(course_m)
   a = 7.221e-06;
   b = -0.004078;
   c = 2.929;
   d = 250;
   course = course_m*1000;
 hauteur = (a*course^3+b*course^2+c*course+d);
end

== matlab function Table_airbus_v2/Ordinateur/MATLAB Function1 ==
  data: ordre3 input; h input; course output
function course = fcn(ordre3,h)
if ordre3==1
   a = -4.511e-8;
   b = 0.0002222;
   c = 0.2369;
   d = -72.39;
else
   a = 0;
   b = 0.0001644;
   c = 0.2604;
   d = -75.41; 
end
course = (a*h^3+b*h^2+c*h+d)/1000;
end

== matlab function Table_airbus_v2/Hacheur 4 Quadrants Unipolaire moyen lev/Hacheur 4 Q/MATLAB Function ==
  data: Rds input; Rd input; Vd input; alpha input; Rhach output; Vhach output
function [Rhach,Vhach]= fcn(Rds,Rd,Vd,alpha)

Rhach = abs(Rds*(1+alpha)+Rd*(1-alpha));

Vhach = Vd*(1-alpha);
end

== matlab function Table_airbus_v2/Hacheur 4 Quadrants Unipolaire moyen Inc/Hacheur 4 Q/MATLAB Function ==
  data: Rds input; Rd input; Vd input; alpha input; Rhach output; Vhach output
function [Rhach,Vhach]= fcn(Rds,Rd,Vd,alpha)

Rhach = abs(Rds*(1+alpha)+Rd*(1-alpha));

Vhach = Vd*(1-alpha);
end

== matlab function Table_airbus_v2/Ordinateur/MATLAB Function2 ==
  data: W_pot input; Course_calcul output; N input
function Course_calcul = fcn(W_pot,N)
Course_calcul = 0.15*double(W_pot)/(2^(N-1)-1);
end

== matlab function Table_airbus_v2/Ordinateur/MATLAB Function3 ==
  data: W_pot input; Course_calcul output; N input
function Course_calcul = fcn(W_pot,N)
Course_calcul = 0.075*double(W_pot)/(2^(N-1)-1);
end

== matlab function Table_airbus_v2/Ordinateur/MATLAB Function4 ==
  data: teta input; course output
function course = fcn(teta)
AD = sqrt(0.08^2+0.135^2);
course = teta*(2*pi/360)*AD;
end

== matlab function Table_airbus_v2/Ordinateur/MATLAB Function5 ==
  data: course input; teta output
function teta = fcn(course)
AD = sqrt(0.08^2+0.135^2);
teta = course*(360/(2*pi))/AD;
end
